simulink model "motor_torque_control"  (R2022a)
settings: Solver=FixedStepAuto  StartTime=0.0  StopTime=0.1  FixedStep=1/500000  RelTol=1e-3
InitFcn:
  | Kt = 0.968; % Nm/A
  | Kv = 1.7103; % V/rad/s
  | L = 2.3e-3; % H
  | R = 2.18; % ohms
  | J = 12e-9 * 12e15; % kgm^2
  | B = 0.0151; % Nm/rad/s
undefined symbols (not defined in the file or in its folder): Down, Up
libraries: eePwmGenerator x1, slpidlib x1
settings Model: Creator=Samvrit  LastModifiedBy=Samvrit

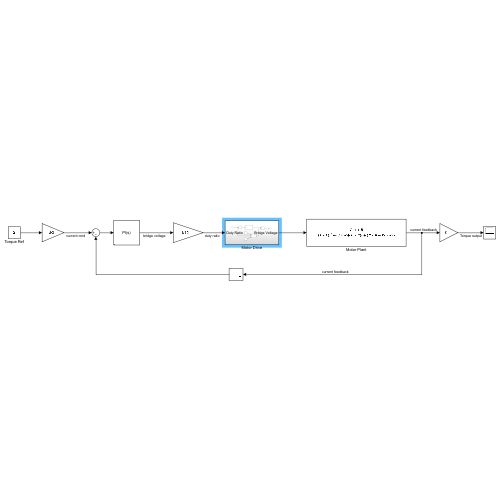
[thumbnail: Simulink's stored preview of the top-level diagram]
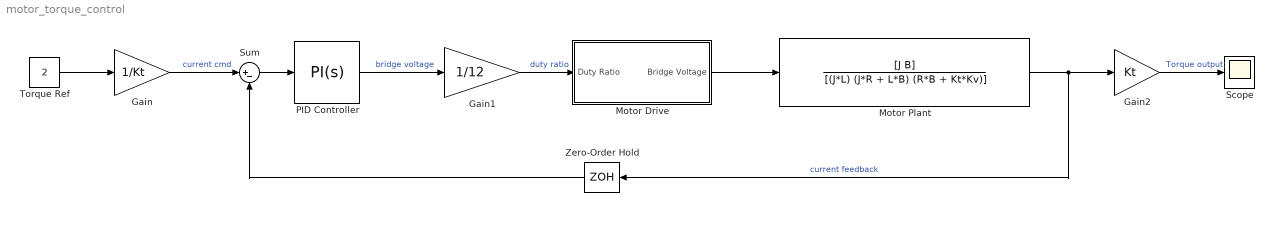
== system motor_torque_control ==
  Gain : Gain  Gain=1/Kt
  Gain1 : Gain  Gain=1/12
  Gain2 : Gain  Gain=Kt
  Motor Drive : Subsystem
  Motor Plant : TransferFcn  Numerator=[J B]  Denominator=[(J*L) (J*R + L*B) (R*B + Kt*Kv)]
  PID Controller : slpidlib/PID Controller  Controller=PI  Form=Parallel  TimeDomain=Continuous-time  UseExternalTs=off  SampleTime=-1  IntegratorMethod=Forward Euler  FilterMethod=Forward Euler  ControllerParametersSource=internal  P=4.4257  I=223640  UseKiTs=off  D=0  N=100  UseFilter=on  TunerSelectOption=Transfer Function Based (PID Tuner App)  InitialConditionSource=internal  InitialConditionForIntegrator=0  InitialConditionForFilter=0  DifferentiatorICPrevScaledInput=0  ExternalReset=none  TrackingMode=off  Kt=1  LimitOutput=off  SatLimitsSource=internal  UpperSaturationLimit=12  LowerSaturationLimit=-12  LinearizeAsGain=on  AntiWindupMode=none  Kb=1  POutMin=[]  POutMax=[]  IOutMin=[]  IOutMax=[]  DOutMin=[]  DOutMax=[]  NOutMin=[]  NOutMax=[]  SumOutMin=[]  SumOutMax=[]  SaturationOutMin=[]  SaturationOutMax=[]  PParamMin=[]  PParamMax=[]  IParamMin=[]  IParamMax=[]  DParamMin=[]  DParamMax=[]  NParamMin=[]  NParamMax=[]  KbParamMin=[]  KbParamMax=[]  KtParamMin=[]  KtParamMax=[]  KbOutMin=[]  KbOutMax=[]  KtOutMin=[]  KtOutMax=[]  IntegratorOutMin=[]  IntegratorOutMax=[]  FilterOutMin=[]  FilterOutMax=[]  SumI1OutMin=[]  SumI1OutMax=[]  SumI2OutMin=[]  SumI2OutMax=[]  SumI3OutMin=[]  SumI3OutMax=[]  SumI4OutMin=[]  SumI4OutMax=[]  SumDOutMin=[]  SumDOutMax=[]  DifferentiatorOutMin=[]  DifferentiatorOutMax=[]  FilterDiffOutCoefMin=[]  FilterDiffOutCoefMax=[]  ReciprocalOutMin=[]  ReciprocalOutMax=[]  SumDenOutMin=[]  SumDenOutMax=[]  SumNumOutMin=[]  SumNumOutMax=[]  DivideOutMin=[]  DivideOutMax=[]  UdiffTsProdOutMin=[]  UdiffTsProdOutMax=[]  NTsProdOutMin=[]  NTsProdOutMax=[]  UintegralTsProdOutMin=[]  UintegralTsProdOutMax=[]  UngainTsProdOutMin=[]  UngainTsProdOutMax=[]  IntegratorContinuousStateAttributes=''  IntegratorStateMustResolveToSignalObject=off  IntegratorRTWStateStorageClass=Auto  FilterContinuousStateAttributes=''  FilterStateMustResolveToSignalObject=off  FilterRTWStateStorageClass=Auto  ParallelPVariant=InternalParameters  IdealPVariant=Disabled  IVariant=InternalParameters  DVariant=Disabled  IntegratorVariant=Continuous  SatVariant=Disabled  AWVariant=Passthrough  PCopyVariant=Disabled  TRVariant=Disabled  FdbkBlocksVariant=Forward  IdealPFdbkVariant=Disabled  SatFdbkVariant=Disabled  DerivativeFilterVariant=Disabled  NVariant=Disabled  NCopyVariant=Disabled_SignalSpec  FilterICVariant=Disabled  IntegratorICVariant=InternalICs  ExternalResetVariant=Disabled  TRSumVariant=Passthrough  SumFdbkVariant=Disabled  SumVariant=Sum_PI  TsampFilterVariant=InternalTs  TsampNgainVariant=Passthrough  TsampIntegralVariant=Passthrough  ExternalSaturationOutDataTypeStr=Inherit: Same as second input  aMode=0
  Scope : Scope
  Sum : Sum  Inputs=|+-
  Torque Ref : Constant  Value=2
  Zero-Order Hold : ZeroOrderHold  SampleTime=1/50000
  wires:
  Motor Plant/1 -> Gain2/1, Zero-Order Hold/1  "current feedback"
  Gain/1 -> Sum/1  "current cmd"
  Torque Ref/1 -> Gain/1
  Sum/1 -> PID Controller/1
  PID Controller/1 -> Gain1/1  "bridge voltage"
  Gain1/1 -> Motor Drive/1(Duty Ratio)  "duty ratio"
  Motor Drive/1(Bridge Voltage) -> Motor Plant/1
  Gain2/1 -> Scope/1  "Torque output"
  Zero-Order Hold/1 -> Sum/2

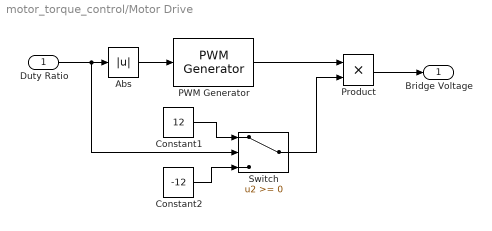
== system motor_torque_control/Motor Drive ==
  Duty Ratio : Inport
  Abs : Abs  SaturateOnIntegerOverflow=off
  Constant1 : Constant  Value=12
  Constant2 : Constant  Value=-12
  PWM Generator : eePwmGenerator/PWM Generator  CarrCount=Up-Down  Tper=1/50000  Tdelay=0  Ts=1/500000
  Product : Product
  Switch : Switch  SaturateOnIntegerOverflow=off  InputSameDT=off
  Bridge Voltage : Outport
  wires:
  Product/1 -> Bridge Voltage/1
  Duty Ratio/1 -> Switch/2, Abs/1
  Abs/1 -> PWM Generator/1
  Constant1/1 -> Switch/1
  Constant2/1 -> Switch/3
  Switch/1 -> Product/2
  PWM Generator/1 -> Product/1
